simulink model "pacemaker_noreqtable"  (R2022a)
settings: Solver=FixedStepAuto  StartTime=0.0  StopTime=10.0  FixedStep=1e-3  RelTol=1e-3  EnableMultiTasking=on
undefined symbols (not defined in the file): A0, A1, D0, D1, D10, D11, D12, D13, D2, D3, D4, D5, D6, D7, D8, D9, PTA0, PTA1, PTA2, PTB2, PTB23, PTB3, PTB9, PTC16, PTC17, PTC2, PTC3, PTC4, PTD0, PTD1, PTD2, PTD3
libraries: frdmk64flib x21, etargetslib x20
settings Model: SimulationMode=external  ExtModeTrigDuration=5  Creator=boran  LastModifiedBy=bryan
settings OptimizationCC: EnhancedBackFolding=on  PassReuseOutputArgsAs=Individual arguments  ZeroExternalMemoryAtStartup=off  ZeroInternalMemoryAtStartup=off  MaxStackSize=64  OptimizeBlockOrder=speed  DifferentSizesBufferReuse=on  OptimizationCustomize=off  EfficientTunableParamExpr=on
settings DebuggingCC: ParameterTunabilityLossMsg=error
settings HardwareCC: ProdBitPerPointer=32  ProdBitPerSizeT=32  ProdBitPerPtrDiffT=32  ProdLargestAtomicInteger=Long  ProdLargestAtomicFloat=Double  ProdWordSize=32  ProdHWDeviceType=ARM Compatible->ARM Cortex
settings ModelReferenceCC: EnableRefExpFcnMdlSchedulingChecks=off
settings SFSimCC: MATLABDynamicMemAlloc=off
settings RTWCC: SystemTargetFile=ert.tlc  HardwareBoard=NXP FRDM-K64F  TLCOptions="-aInlineSetEventsForThisBaseRateFcn=TLC_FALSE -aSuppressMultiTaskScheduler=TLC_FALSE  -aRateBasedStepFcn=0"  TemplateMakefile=ert_default_tmf  Toolchain=GNU Tools for ARM Embedded Processors
settings CodeAppCC: ForceParamTrailComments=on  IgnoreCustomStorageClasses=off  OperatorAnnotations=on  SimulinkDataObjDesc=on  SFDataObjDesc=on  InsertBlockDesc=on
settings ERTTargetCC: ExtModeTransport=4  ExtModeMexFile=sendToCommService

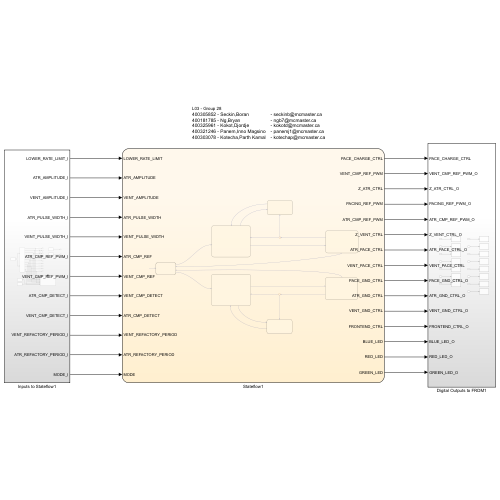
[thumbnail: Simulink's stored preview of the top-level diagram]
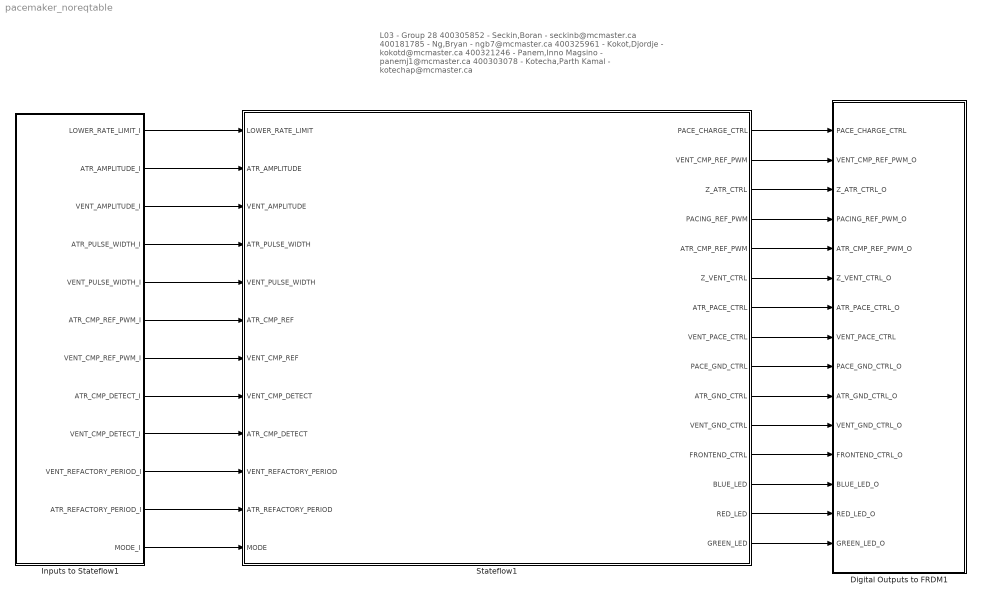
== system pacemaker_noreqtable ==
  note: L03 - Group 28
      | 400305852 - Seckin,Boran - seckinb@mcmaster.ca
      | 400181785 - Ng,Bryan - ngb7@mcmaster.ca
      | 400325961 - Kokot,Djordje - kokotd@mcmaster.ca
      | 400321246 - Panem,Inno Magsino - panemj1@mcmaster.ca
      | 400303078 - Kotecha,Parth Kamal - kotechap@mcmaster.ca
  Digital Outputs to FRDM1 : Subsystem
  Inputs to Stateflow1 : Subsystem
  Stateflow1 : Stateflow chart  TreatAsAtomicUnit=on
      settings: PortSchema="{\"entries\":[{\"content\":{\"sides\":[{\"content\":{\"connectorIds\":[\"In1\",\"In2\",\"In5\",\"In3\",\"In6\",\"In8\",\"In7\",\"In9\",\"In10\",\"In11\",\"In12\",\"In4\"]},\"type\":\"ConnectorPlacement.EquallySpacedRectSide\",\"uuid\":\"52f736ed-aeb0-4856-87f7-b93590276344\"},{\"content\":{\"connectorIds\":[\"Out1\",\"Out12\",\"Out6\",\"Out2\",\"Out14\",\"Out7\",\"Out4\",\"Out5\",\"Out3\",\"Out8\",\"Out9\",\"Out13\",\"Out11\",\"Out10\",\"Out15\"],\"side\":\"RIGHT\"},\"type\":\"ConnectorPlacement.EquallySpacedRectSide\",\"uuid\":\"db458224-1bef-40aa-b553-5edb14e40add\"},{\"content\":{\"connectorIds\":[],\"side\":\"TOP\"},\"type\":\"ConnectorPlacement.EquallySpacedRectSide\",\"uuid\":\"203d36c3-44b0-4680-9041-c599d24a16de\"}]},\"type\":\"ConnectorPlacement.EquallySpacedConnector\",\"uuid\":\"0b64f242-bdb6-4003-8677-cbb5c211967e\"}],\"packageUris\":[\"http://schema.mathworks.com/mf0/Connector/R2020b\"],\"version\":\"1.0\"}"
  wires:
  Inputs to Stateflow1/3(VENT_AMPLITUDE_I) -> Stateflow1/5(VENT_AMPLITUDE)
  Stateflow1/10(RED_LED) -> Digital Outputs to FRDM1/14(RED_LED_O)
  Stateflow1/11(BLUE_LED) -> Digital Outputs to FRDM1/13(BLUE_LED_O)
  Stateflow1/1(PACE_CHARGE_CTRL) -> Digital Outputs to FRDM1/1(PACE_CHARGE_CTRL)
  Stateflow1/14(ATR_CMP_REF_PWM) -> Digital Outputs to FRDM1/5(ATR_CMP_REF_PWM_O)
  Stateflow1/5(VENT_PACE_CTRL) -> Digital Outputs to FRDM1/8(VENT_PACE_CTRL)
  Stateflow1/15(GREEN_LED) -> Digital Outputs to FRDM1/15(GREEN_LED_O)
  Inputs to Stateflow1/2(ATR_AMPLITUDE_I) -> Stateflow1/2(ATR_AMPLITUDE)
  Inputs to Stateflow1/9(VENT_CMP_DETECT_I) -> Stateflow1/10(ATR_CMP_DETECT)
  Stateflow1/6(Z_ATR_CTRL) -> Digital Outputs to FRDM1/3(Z_ATR_CTRL_O)
  Inputs to Stateflow1/11(ATR_REFACTORY_PERIOD_I) -> Stateflow1/12(ATR_REFACTORY_PERIOD)
  Stateflow1/2(PACING_REF_PWM) -> Digital Outputs to FRDM1/4(PACING_REF_PWM_O)
  Inputs to Stateflow1/6(ATR_CMP_REF_PWM_I) -> Stateflow1/8(ATR_CMP_REF)
  Stateflow1/13(FRONTEND_CTRL) -> Digital Outputs to FRDM1/12(FRONTEND_CTRL_O)
  Stateflow1/7(Z_VENT_CTRL) -> Digital Outputs to FRDM1/6(Z_VENT_CTRL_O)
  Inputs to Stateflow1/10(VENT_REFACTORY_PERIOD_I) -> Stateflow1/11(VENT_REFACTORY_PERIOD)
  Inputs to Stateflow1/7(VENT_CMP_REF_PWM_I) -> Stateflow1/7(VENT_CMP_REF)
  Inputs to Stateflow1/4(ATR_PULSE_WIDTH_I) -> Stateflow1/3(ATR_PULSE_WIDTH)
  Inputs to Stateflow1/12(MODE_I) -> Stateflow1/4(MODE)
  Inputs to Stateflow1/1(LOWER_RATE_LIMIT_I) -> Stateflow1/1(LOWER_RATE_LIMIT)
  Stateflow1/3(PACE_GND_CTRL) -> Digital Outputs to FRDM1/9(PACE_GND_CTRL_O)
  Inputs to Stateflow1/8(ATR_CMP_DETECT_I) -> Stateflow1/9(VENT_CMP_DETECT)
  Stateflow1/9(VENT_GND_CTRL) -> Digital Outputs to FRDM1/11(VENT_GND_CTRL_O)
  Stateflow1/12(VENT_CMP_REF_PWM) -> Digital Outputs to FRDM1/2(VENT_CMP_REF_PWM_O)
  Stateflow1/8(ATR_GND_CTRL) -> Digital Outputs to FRDM1/10(ATR_GND_CTRL_O)
  Inputs to Stateflow1/5(VENT_PULSE_WIDTH_I) -> Stateflow1/6(VENT_PULSE_WIDTH)
  Stateflow1/4(ATR_PACE_CTRL) -> Digital Outputs to FRDM1/7(ATR_PACE_CTRL_O)

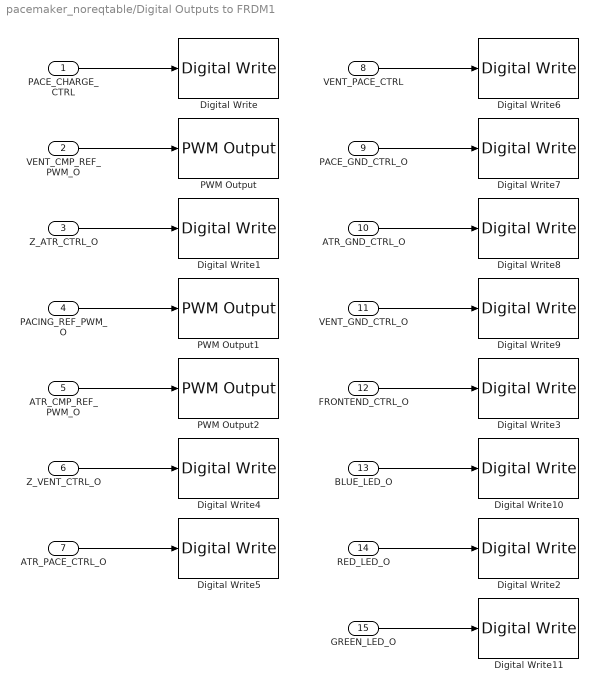
== system pacemaker_noreqtable/Digital Outputs to FRDM1 ==
  PACE_CHARGE_CTRL : Inport
  VENT_CMP_REF_PWM_O : Inport  Port=2
  Z_ATR_CTRL_O : Inport  Port=3
  PACING_REF_PWM_O : Inport  Port=4
  ATR_CMP_REF_PWM_O : Inport  Port=5
  Z_VENT_CTRL_O : Inport  Port=6
  ATR_PACE_CTRL_O : Inport  Port=7
  VENT_PACE_CTRL : Inport  Port=8
  PACE_GND_CTRL_O : Inport  Port=9
  ATR_GND_CTRL_O : Inport  Port=10
  VENT_GND_CTRL_O : Inport  Port=11
  FRONTEND_CTRL_O : Inport  Port=12
  BLUE_LED_O : Inport  Port=13
  RED_LED_O : Inport  Port=14
  GREEN_LED_O : Inport  Port=15
  Digital Write : frdmk64flib/Digital Write  Whichpin=PTB9 (D2)
  Digital Write1 : frdmk64flib/Digital Write  Whichpin=PTB23 (D4)
  Digital Write10 : frdmk64flib/Digital Write  Whichpin=BLUE_LED
  Digital Write11 : frdmk64flib/Digital Write  Whichpin=GREEN_LED
  Digital Write2 : frdmk64flib/Digital Write  Whichpin=RED_LED
  Digital Write3 : frdmk64flib/Digital Write  Whichpin=PTD1 (D13)
  Digital Write4 : frdmk64flib/Digital Write  Whichpin=PTC3 (D7)
  Digital Write5 : frdmk64flib/Digital Write  Whichpin=PTA0 (D8)
  Digital Write6 : frdmk64flib/Digital Write  Whichpin=PTC4 (D9)
  Digital Write7 : frdmk64flib/Digital Write  Whichpin=PTD0 (D10)
  Digital Write8 : frdmk64flib/Digital Write  Whichpin=PTD2 (D11)
  Digital Write9 : frdmk64flib/Digital Write  Whichpin=PTD3 (D12)
  PWM Output : frdmk64flib/PWM Output  Whichpin=PTA1 (D3)  InitialFrequency=2000  InitialDutyCycle=0
  PWM Output1 : frdmk64flib/PWM Output  Whichpin=PTA2 (D5)  InitialFrequency=2000  InitialDutyCycle=0
  PWM Output2 : frdmk64flib/PWM Output  Whichpin=PTC2 (D6)  InitialFrequency=2000  InitialDutyCycle=0
  wires:
  ATR_GND_CTRL_O/1 -> Digital Write8/1
  PACE_GND_CTRL_O/1 -> Digital Write7/1
  VENT_PACE_CTRL/1 -> Digital Write6/1
  ATR_PACE_CTRL_O/1 -> Digital Write5/1
  VENT_CMP_REF_PWM_O/1 -> PWM Output/1
  PACE_CHARGE_CTRL/1 -> Digital Write/1
  ATR_CMP_REF_PWM_O/1 -> PWM Output2/1
  Z_VENT_CTRL_O/1 -> Digital Write4/1
  Z_ATR_CTRL_O/1 -> Digital Write1/1
  VENT_GND_CTRL_O/1 -> Digital Write9/1
  FRONTEND_CTRL_O/1 -> Digital Write3/1
  BLUE_LED_O/1 -> Digital Write10/1
  PACING_REF_PWM_O/1 -> PWM Output1/1
  RED_LED_O/1 -> Digital Write2/1
  GREEN_LED_O/1 -> Digital Write11/1

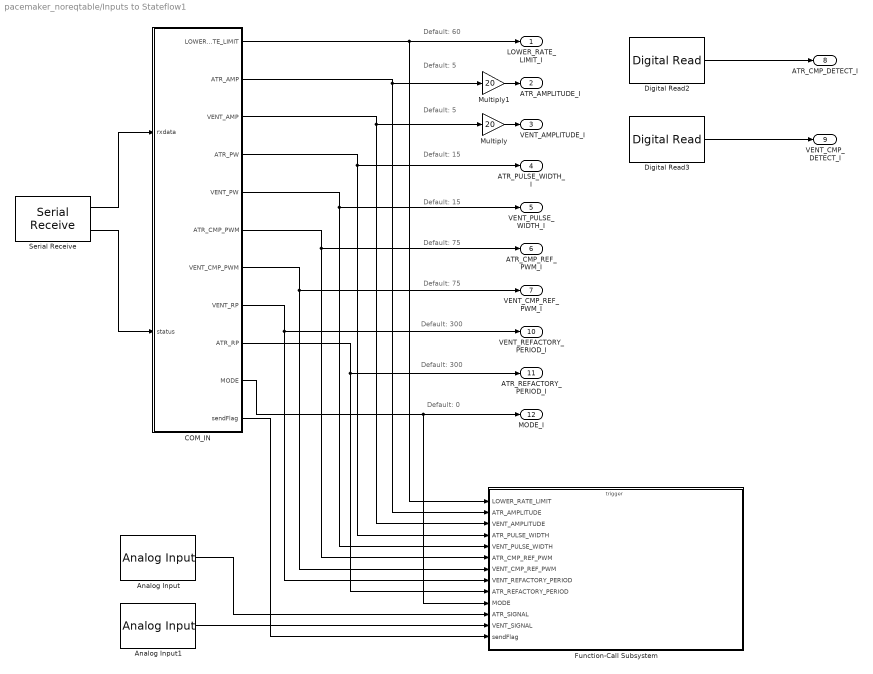
== system pacemaker_noreqtable/Inputs to Stateflow1 ==
  note: Default: 60
  note: Default: 5
  note: Default: 5
  note: Default: 15
  note: Default: 15
  note: Default: 75
  note: Default: 75
  note: Default: 300
  note: Default: 300
  note: Default: 0
  Analog Input : frdmk64flib/Analog Input  Whichpin=PTB2 (A0)  SampleTime=-1
  Analog Input1 : frdmk64flib/Analog Input  Whichpin=PTB3 (A1)  SampleTime=-1
  COM_IN : Stateflow chart  TreatAsAtomicUnit=on
  Digital Read2 : frdmk64flib/Digital Read  Whichpin=PTC17 (D1)  SampleTime=-1
  Digital Read3 : frdmk64flib/Digital Read  Whichpin=PTC16 (D0)  SampleTime=-1
  Function-Call Subsystem : Subsystem  TreatAsAtomicUnit=on
  Multiply : Gain  Gain=20
  Multiply1 : Gain  Gain=20
  Serial Receive : frdmk64flib/Serial Receive  SCIModule=0  Baudrate=uint32(9600)  Parity=None  StopBits=1  HardwareFlowControl=None  ByteOrder=LittleEndian  DataType=uint8  DataLength=25  BlockingMode=off  OutputStatus=on  SampleTime=-1
  LOWER_RATE_LIMIT_I : Outport
  ATR_AMPLITUDE_I : Outport  Port=2
  VENT_AMPLITUDE_I : Outport  Port=3
  ATR_PULSE_WIDTH_I : Outport  Port=4
  VENT_PULSE_WIDTH_I : Outport  Port=5
  ATR_CMP_REF_PWM_I : Outport  Port=6
  VENT_CMP_REF_PWM_I : Outport  Port=7
  ATR_CMP_DETECT_I : Outport  Port=8
  VENT_CMP_DETECT_I : Outport  Port=9
  VENT_REFACTORY_PERIOD_I : Outport  Port=10
  ATR_REFACTORY_PERIOD_I : Outport  Port=11
  MODE_I : Outport  Port=12
  wires:
  Digital Read2/1 -> ATR_CMP_DETECT_I/1
  COM_IN/7(VENT_CMP_PWM) -> Function-Call Subsystem/7(VENT_CMP_REF_PWM), VENT_CMP_REF_PWM_I/1
  Digital Read3/1 -> VENT_CMP_DETECT_I/1
  COM_IN/9(ATR_RP) -> Function-Call Subsystem/9(ATR_REFACTORY_PERIOD), ATR_REFACTORY_PERIOD_I/1
  COM_IN/6(ATR_CMP_PWM) -> Function-Call Subsystem/6(ATR_CMP_REF_PWM), ATR_CMP_REF_PWM_I/1
  COM_IN/1(LOWER_RATE_LIMIT) -> Function-Call Subsystem/1(LOWER_RATE_LIMIT), LOWER_RATE_LIMIT_I/1
  COM_IN/2(ATR_AMP) -> Function-Call Subsystem/2(ATR_AMPLITUDE), Multiply1/1
  COM_IN/3(VENT_AMP) -> Function-Call Subsystem/3(VENT_AMPLITUDE), Multiply/1
  COM_IN/4(ATR_PW) -> Function-Call Subsystem/4(ATR_PULSE_WIDTH), ATR_PULSE_WIDTH_I/1
  COM_IN/5(VENT_PW) -> Function-Call Subsystem/5(VENT_PULSE_WIDTH), VENT_PULSE_WIDTH_I/1
  COM_IN/10(MODE) -> MODE_I/1, Function-Call Subsystem/10(MODE)
  COM_IN/8(VENT_RP) -> Function-Call Subsystem/8(VENT_REFACTORY_PERIOD), VENT_REFACTORY_PERIOD_I/1
  Serial Receive/1 -> COM_IN/1(rxdata)
  Serial Receive/2 -> COM_IN/2(status)
  Multiply/1 -> VENT_AMPLITUDE_I/1
  Multiply1/1 -> ATR_AMPLITUDE_I/1
  Analog Input/1 -> Function-Call Subsystem/11(ATR_SIGNAL)
  Analog Input1/1 -> Function-Call Subsystem/12(VENT_SIGNAL)
  COM_IN/11(sendFlag) -> Function-Call Subsystem/13(sendFlag)

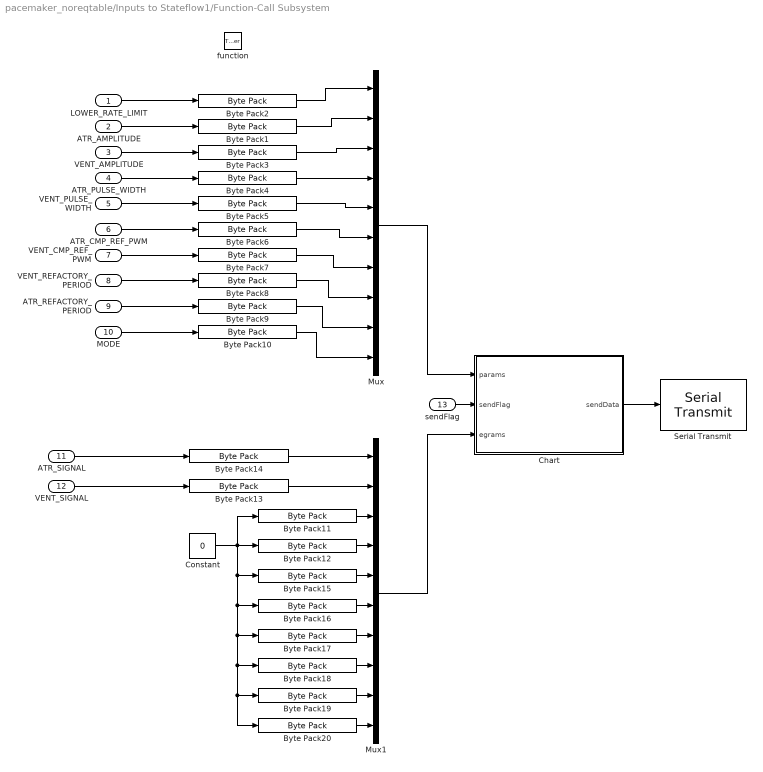
== system pacemaker_noreqtable/Inputs to Stateflow1/Function-Call Subsystem ==
  LOWER_RATE_LIMIT : Inport
  ATR_AMPLITUDE : Inport  Port=2
  VENT_AMPLITUDE : Inport  Port=3
  ATR_PULSE_WIDTH : Inport  Port=4
  VENT_PULSE_WIDTH : Inport  Port=5
  ATR_CMP_REF_PWM : Inport  Port=6
  VENT_CMP_REF_PWM : Inport  Port=7
  VENT_REFACTORY_PERIOD : Inport  Port=8
  ATR_REFACTORY_PERIOD : Inport  Port=9
  MODE : Inport  Port=10
  ATR_SIGNAL : Inport  Port=11
  VENT_SIGNAL : Inport  Port=12
  sendFlag : Inport  Port=13
  function : TriggerPort  TriggerType=function-call  IsSimulinkFunction=on  FunctionName=send_params  VariantControl=(inherit)
  Byte Pack{1..20} (20 alike) : etargetslib/Byte Pack  datatypes={'double'}  byteAlign=1
  Chart : Stateflow chart  TreatAsAtomicUnit=on
  Constant : Constant  Value=0
  Mux : Mux  Inputs=10
  Mux1 : Mux  Inputs=10
  Serial Transmit : frdmk64flib/Serial Transmit  SCIModule=0  Baudrate=uint32(9600)  Parity=None  StopBits=1  HardwareFlowControl=None  ByteOrder=LittleEndian  BlockingMode=on  OutputStatus=off
  wires:
  LOWER_RATE_LIMIT/1 -> Byte Pack2/1
  MODE/1 -> Byte Pack10/1
  Byte Pack1/1 -> Mux/2
  Byte Pack2/1 -> Mux/1
  Byte Pack3/1 -> Mux/3
  Byte Pack4/1 -> Mux/4
  Byte Pack5/1 -> Mux/5
  Byte Pack6/1 -> Mux/6
  Byte Pack7/1 -> Mux/7
  Byte Pack8/1 -> Mux/8
  Byte Pack9/1 -> Mux/9
  Byte Pack10/1 -> Mux/10
  ATR_REFACTORY_PERIOD/1 -> Byte Pack9/1
  VENT_REFACTORY_PERIOD/1 -> Byte Pack8/1
  VENT_CMP_REF_PWM/1 -> Byte Pack7/1
  ATR_CMP_REF_PWM/1 -> Byte Pack6/1
  VENT_PULSE_WIDTH/1 -> Byte Pack5/1
  ATR_PULSE_WIDTH/1 -> Byte Pack4/1
  VENT_AMPLITUDE/1 -> Byte Pack3/1
  ATR_AMPLITUDE/1 -> Byte Pack1/1
  VENT_SIGNAL/1 -> Byte Pack13/1
  ATR_SIGNAL/1 -> Byte Pack14/1
  Byte Pack13/1 -> Mux1/2
  Byte Pack14/1 -> Mux1/1
  Mux/1 -> Chart/1(params)
  Mux1/1 -> Chart/3(egrams)
  Chart/1(sendData) -> Serial Transmit/1
  sendFlag/1 -> Chart/2(sendFlag)
  Constant/1 -> Byte Pack20/1, Byte Pack19/1, Byte Pack18/1, Byte Pack17/1, Byte Pack16/1, Byte Pack15/1, Byte Pack11/1, Byte Pack12/1
  Byte Pack20/1 -> Mux1/10
  Byte Pack19/1 -> Mux1/9
  Byte Pack18/1 -> Mux1/8
  Byte Pack17/1 -> Mux1/7
  Byte Pack16/1 -> Mux1/6
  Byte Pack15/1 -> Mux1/5
  Byte Pack12/1 -> Mux1/4
  Byte Pack11/1 -> Mux1/3

== stateflow chart pacemaker_noreqtable/Inputs to Stateflow1/Function-Call Subsystem/Chart ==
  state send_params
    entry:
    sendData = params;
  state INITIAL
  state send_egram
    entry:
    sendData = egrams;
  send_params -> INITIAL
  INITIAL -> send_params [order 1] : [sendFlag==hex2dec('20')]
  (default) -> INITIAL
  send_egram -> INITIAL
  INITIAL -> send_egram [order 2] : [sendFlag==hex2dec('30')]
  data: params input; sendFlag input; egrams input; sendData output

== stateflow chart pacemaker_noreqtable/Inputs to Stateflow1/COM_IN ==
  state SET_PARAM
    entry:
    LOWER_RATE_LIMIT = double(typecast(rxdata(2:3), 'uint16'));
    ATR_AMP = double(typecast(rxdata(4:7), 'single'));
    VENT_AMP = double(typecast(rxdata(8:11), 'single'));
    ATR_PW = double(typecast(rxdata(12:13), 'uint16'));
    VENT_PW = double(typecast(rxdata(14:15), 'uint16'));
    ATR_CMP_PWM = double(typecast(rxdata(16:17), 'uint16'));
    VENT_CMP_PWM = double(typecast(rxdata(18:19), 'uint16'));
    VENT_RP = double(typecast(rxdata(20:21), 'uint16'));
    ATR_RP = double(typecast(rxdata(22:23), 'uint16'));
    MODE = double(typecast(rxdata(24:25), 'uint16'));
  state INITIAL
    entry:
    LOWER_RATE_LIMIT = double(60);
    ATR_AMP = double(5);
    VENT_AMP = double(5);
    ATR_PW = double(15);
    VENT_PW = double(15);
    ATR_CMP_PWM = double(75);
    VENT_CMP_PWM = double(75);
    VENT_RP = double(300);
    ATR_RP = double(300);
    MODE = double(0);
  state STANDBY
    entry:
  state Send_PARAMS
    entry:
    sendFlag = rxdata(2);
    send_params();
  state Send_EGRAM
    entry:
    sendFlag = rxdata(2);
    send_params();
  SET_PARAM -> STANDBY
  (default) -> INITIAL
  (junction 55) -> SET_PARAM [order 2] : [rxdata(2)==hex2dec('10')]
  (junction 14) -> STANDBY [order 1]
  INITIAL -> STANDBY
  STANDBY -> (junction 14) : [status==0]
  (junction 14) -> (junction 55) [order 2] : [rxdata(1)==hex2dec(10)]
  (junction 55) -> Send_EGRAM [order 1] : [rxdata(2)==hex2dec('20')]
  (junction 55) -> Send_PARAMS [order 3] : [rxdata(2)==hex2dec('30')]
  Send_EGRAM -> STANDBY
  Send_PARAMS -> STANDBY
  data: rxdata input uint8; status input uint8; LOWER_RATE_LIMIT output; ATR_AMP output; VENT_AMP output; ATR_PW output; VENT_PW output; ATR_CMP_PWM output; VENT_CMP_PWM output; VENT_RP output; ATR_RP output; MODE output; sendFlag output

== stateflow chart pacemaker_noreqtable/Stateflow1 ==
  note: A atrium pace is sensed. This pace is either induced by the pacemaker (AOO_PACE) or it is a natural heart beat. Nevertheless, the current AOO_PACE is inhibited until the next cycle.
      |
      | The color of the LED will be green if natural ventricle beat is sensed and yellow (red + green) if atrium is paced.
  note: Wait for the specified amount of refactory time to not sens the same heartbeat signal multiple times. Add this wait time to the delta, so that it does not affect the next cycle.
  state AAI_SENSED
    entry:
    GREEN_LED = true;
  note: Charge state sets the compare reference value for sensing (in case that AAI is activated), disables all pace controls, sets the pace amplitude (required charge for C22) for the atrium and starts charging C22.
      | Additionally, it discharges C21 via atrium by enabling pace ground, disabling both impedence controls, disabling ventricle ground control and enabling atrium ground control.
      | It resets all the LED signals to turn it off.
  note: Pace state discharges C22 by disabling pace charge control, enabling pace ground control, disabling ventricle pace and ground controls, disabling both impedence controls, disabling atrium ground control and enabling atrium pace control.
      | It also turns on red led to show the atrium is paced.
  note: Natural heartbeat is detected, inhibit the pace. Reset the delta for the next cycle.
  note: AAI
  state AOO_CHARGE
    entry:
    % SET CMP REF for sensing
    ATR_CMP_REF_PWM = ATR_CMP_REF;
    % CHARGE C22
    ATR_PACE_CTRL = false;
    VENT_PACE_CTRL = false;
    PACING_REF_PWM = ATR_AMPLITUDE;
    PACE_CHARGE_CTRL = true;
    % DISCHARGE C21
    PACE_GND_CTRL = true;
    Z_ATR_CTRL = false;
    Z_VENT_CTRL = false;
    VENT_GND_CTRL = false;
    ATR_GND_CTRL = true;
    RED_LED = false;
    BLUE_LED = false;
    GREEN_LED = false;
  note: Wait for the pulse to be delivered. Set the delta to the length of the pulse, so that it is subtracted from the next wait duration.
  state AOO_PACE
    entry:
    % DISCHARGE C22
    PACE_CHARGE_CTRL = false;
    PACE_GND_CTRL = true;
    VENT_PACE_CTRL = false;
    VENT_GND_CTRL = false;
    Z_ATR_CTRL = false;
    Z_VENT_CTRL = false;
    ATR_GND_CTRL = false;
    ATR_PACE_CTRL = true;
    RED_LED = true;
  note: AOO
  note: AOO (0) and AAI (1)
  note: Wait for the lower rate limit specified minus the extra time already spent waiting during the previous states (ATR_Delta).
  state START
    entry:
    FRONTEND_CTRL = true;
    ATR_Delta = 0;
    VENT_Delta = 0;
  note: Return to start if the mode has changed.
  state VOO_CHARGE
    entry:
    % SET CMP REF for sensing
    VENT_CMP_REF_PWM = VENT_CMP_REF;
    % CHARGE C22
    ATR_PACE_CTRL = false;
    VENT_PACE_CTRL = false;
    PACING_REF_PWM = VENT_AMPLITUDE;
    PACE_CHARGE_CTRL = true;
    % DISCHARGE C21
    PACE_GND_CTRL = true;
    Z_ATR_CTRL = false;
    Z_VENT_CTRL = false;
    ATR_GND_CTRL = false;
    VENT_GND_CTRL = true;
    RED_LED = false;
    BLUE_LED = false;
    GREEN_LED = false;
  note: Entry state enables frontend control (in case sensing is used) and resets both delta values.
  note: Wait for the lower rate limit specified minus the extra time already spent waiting during the previous states (VENT_Delta).
  state VOO_PACE
    entry:
    % DISCHARGE C22
    PACE_CHARGE_CTRL = false;
    PACE_GND_CTRL = true;
    ATR_PACE_CTRL = false;
    ATR_GND_CTRL = false;
    Z_ATR_CTRL = false;
    Z_VENT_CTRL = false;
    VENT_GND_CTRL = false;
    VENT_PACE_CTRL = true;
    BLUE_LED = true;
  note: VOO (2) and VVI (3)
  note: VOO
  note: Wait for the pulse to be delivered. Set the delta to the length of the pulse, so that it is subtracted from the next wait duration.
  note: Pace state discharges C22 by disabling pace charge control, enabling pace ground control, disabling atrium pace and ground controls, disabling both impedence controls, disabling ventricle ground control and enabling ventricle pace control.
      | It also turns on blue led to show the ventricle is paced.
  note: VVI
  note: Charge state sets the compare reference value for sensing (in case that VVI is activated), disables all pace controls, sets the pace amplitude (required charge for C22) for the ventricle and starts charging C22.
      | Additionally, it discharges C21 via ventricle by enabling pace ground, disabling both impedence controls, disabling atrium ground control and enabling ventricle ground control.
      | It resets all the LED signals to turn it off.
  note: Natural heartbeat is detected, inhibit the pace. Reset the delta for the next cycle.
  state VVI_SENSED
    entry:
    GREEN_LED = true;
  note: A ventricular pace is sensed. This pace is either induced by the pacemaker (VOO_PACE) or it is a natural heart beat. Nevertheless, the current VOO_PACE is inhibited until the next cycle.
      |
      | The color of the LED will be green if natural ventricle beat is sensed and cyan (blue + green) if ventricle is paced.
  note: Wait for the specified amount of refactory time to not sens the same heartbeat signal multiple times. Add this wait time to the delta, so that it does not affect the next cycle.
  AAI_SENSED -> AOO_CHARGE : after(ATR_REFACTORY_PERIOD, msec)
      | {ATR_Delta = ATR_Delta + ATR_REFACTORY_PERIOD}
  AOO_CHARGE -> AAI_SENSED [order 2] : [MODE == 1 && ATR_CMP_DETECT]
      | {ATR_Delta = 0}
  (junction 69) -> AAI_SENSED [order 1] : [MODE == 1]
  (junction 69) -> AOO_CHARGE [order 2] : [MODE == 0]
  AOO_PACE -> (junction 69) [order 1] : after(ATR_PULSE_WIDTH, msec)
      | {ATR_Delta = ATR_PULSE_WIDTH}
  START -> AOO_CHARGE [order 1] : [MODE == 0 | MODE == 1]
  AOO_CHARGE -> AOO_PACE [order 1] : after([60000/LOWER_RATE_LIMIT] - ATR_Delta, msec)
  AOO_PACE -> START [order 2] : [MODE ~= 0 && MODE ~= 1]
  (default) -> START
  VOO_PACE -> START [order 2] : [MODE ~= 2 && MODE ~= 3]
  START -> VOO_CHARGE [order 2] : [MODE == 2 | MODE == 3]
  VOO_CHARGE -> VOO_PACE [order 1] : after([60000/LOWER_RATE_LIMIT] - VENT_Delta, msec)
  (junction 59) -> VOO_CHARGE [order 1] : [MODE == 2]
  VOO_PACE -> (junction 59) [order 1] : after(VENT_PULSE_WIDTH, msec)
      | {VENT_Delta = VENT_PULSE_WIDTH}
  (junction 59) -> VVI_SENSED [order 2] : [MODE == 3]
  VVI_SENSED -> VOO_CHARGE : after(VENT_REFACTORY_PERIOD, msec)
      | {VENT_Delta = VENT_Delta + VENT_REFACTORY_PERIOD}
  VOO_CHARGE -> VVI_SENSED [order 2] : [MODE == 3 && VENT_CMP_DETECT]
      | {VENT_Delta = 0}
  data: PACE_CHARGE_CTRL output; PACING_REF_PWM output; PACE_GND_CTRL output; ATR_PACE_CTRL output; LOWER_RATE_LIMIT input; ATR_AMPLITUDE input; ATR_PULSE_WIDTH input; VENT_PACE_CTRL output; Z_ATR_CTRL output; Z_VENT_CTRL output; ATR_GND_CTRL output; VENT_GND_CTRL output; RED_LED output; MODE input; VENT_AMPLITUDE input; BLUE_LED output; VENT_PULSE_WIDTH input; VENT_CMP_REF_PWM output; VENT_CMP_REF input; FRONTEND_CTRL output; ATR_CMP_REF_PWM output; ATR_CMP_REF input; VENT_CMP_DETECT input; ATR_CMP_DETECT input; VENT_REFACTORY_PERIOD input; ATR_REFACTORY_PERIOD input; VENT_Delta local; ATR_Delta local; GREEN_LED output
